simulink library "soar_interp"  (R2018b)
settings: Solver=VariableStepAuto  StartTime=0.0  StopTime=10.0  RelTol=1e-3
undefined symbols (not defined in the file): soarParams
settings Model: Creator=Taylor  LastModifiedBy=Nick's PC

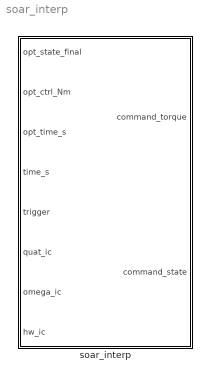
== system soar_interp ==
  soar_interp : Subsystem

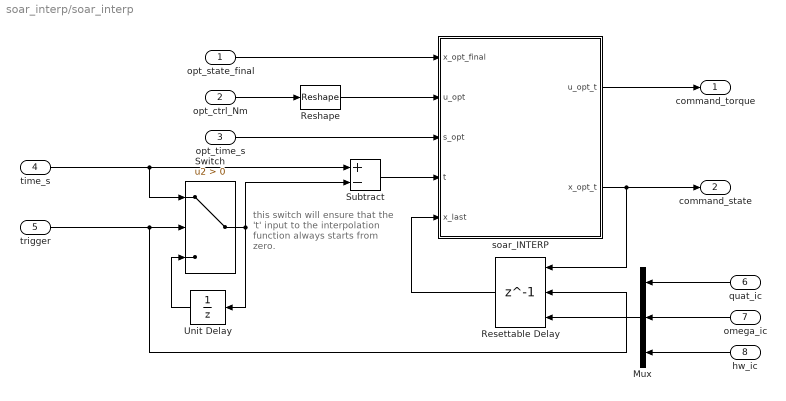
== system soar_interp/soar_interp ==
  note: this switch will ensure that the 't'
      | input to the interpolation function
      | always starts from zero.
  opt_state_final : Inport
  opt_ctrl_Nm : Inport  Port=2
  opt_time_s : Inport  Port=3
  time_s : Inport  Port=4
  trigger : Inport  Port=5
  quat_ic : Inport  Port=6
  omega_ic : Inport  Port=7
  hw_ic : Inport  Port=8
  Mux : Mux  Inputs=[4 3 3]
  Resettable Delay : Delay  DelayLength=1  InitialConditionSource=Input port  ExternalReset=Rising
      settings: InputPortMap=u0,r5,p4
  Reshape : Reshape  OutputDimensionality=Customize  OutputDimensions=[3,soarParams.N]
  Subtract : Sum  Inputs=+-
  Switch : Switch  Criteria=u2 > Threshold
  Unit Delay : UnitDelay  SampleTime=-1
  soar_INTERP : MATLAB Function  TreatAsAtomicUnit=on
  command_torque : Outport
  command_state : Outport  Port=2
  wires:
  omega_ic/1 -> Mux/2
  Mux/1 -> Resettable Delay/3
  Subtract/1 -> soar_INTERP/4(t)
  Resettable Delay/1 -> soar_INTERP/5(x_last)
  Unit Delay/1 -> Switch/3
  opt_state_final/1 -> soar_INTERP/1(x_opt_final)
  Switch/1 -> Unit Delay/1, Subtract/2
  Reshape/1 -> soar_INTERP/2(u_opt)
  trigger/1 -> Resettable Delay/2, Switch/2
  time_s/1 -> Switch/1, Subtract/1
  opt_ctrl_Nm/1 -> Reshape/1
  opt_time_s/1 -> soar_INTERP/3(s_opt)
  soar_INTERP/1(u_opt_t) -> command_torque/1
  soar_INTERP/2(x_opt_t) -> command_state/1, Resettable Delay/1
  quat_ic/1 -> Mux/1
  hw_ic/1 -> Mux/3

== matlab function soar_interp/soar_INTERP ==
  data: u_opt_t output size=3; x_opt_final input size=10; x_opt_t output size=10; u_opt input; s_opt input size=1; t input size=1; x_last input size=10; soarParams parameter
function [u_opt_t,x_opt_t] = soar_INTERP(x_opt_final,u_opt,s_opt,t,x_last,soarParams)
%SOAR_INTERP
%
% This function will interpolate the optimal solution from SOAR given the
% time t. Time t is assumed to represent the time SINCE the optimizer was
% called by flight software (necessitating the switch outside of this
% function). One RK4 step is performed to interpolate the state, while the
% control is interpolated using affine interpolation.
%
% T. Reynolds -- RAIN LAB

%#codegen

% parameters
N  = soarParams.N;
Ns = 10;
ut = linspace(0,s_opt,N);
k  = sum(t>ut); % current time interval
if (k==0); k = 1; end
J  = soarParams.inertia; % kg m2

% Output final state and ZERO feedforward control if we are beyond the 
% final maneuver time
if ((s_opt>eps)&&(t>=s_opt))
    u_opt_t = zeros(3,1);
    x_opt_t = [ x_opt_final(1:4); J\x_opt_final(5:7); x_opt_final(8:10) ];
    return;
end

% Otherwise integrate to current state and interpolate for current control
if ((k>0) && (s_opt>eps))
    dt = soarParams.sample_time_s/Ns;
    
    % step integrator for feedforward state x_opt_t
    x_opt_t = rk4_step(t,x_last,u_opt,ut,J,dt,Ns);

    % interpolate for feedforward control u_opt_t
    u_opt_t = zeros(3,1);
    for i = 1:3
        if t > ut(end) || t < ut(1)
            u_opt_t = zeros(3,1);
        else
            u_opt_t(i) = interp1(ut,u_opt(i,:),t,'linear');
        end
    end
else
    % this case happens when the optimizer has not yet been called
    u_opt_t = zeros(3,1);
    x_opt_t = x_last;
end

end % soar_interp

%%%%%%%%%%%%%%%%%%%%%%%%%%%%%%%%%%%%%%%%%%%%%%%%%%%%%%%%%%%%%%%%%%%%%%%%%%%
%%%%%%%%%%%%%%%%%%%%%%%%%%%% SUPPORT FUNCTIONS %%%%%%%%%%%%%%%%%%%%%%%%%%%%
%%%%%%%%%%%%%%%%%%%%%%%%%%%%%%%%%%%%%%%%%%%%%%%%%%%%%%%%%%%%%%%%%%%%%%%%%%%

function x = rk4_step(t,x,u,ut,J,h,Ns)

for ii = 1:Ns
    k1 = deriv(t     ,x      ,u,ut,J);
    k2 = deriv(t+h/2,x+h/2*k1,u,ut,J);
    k3 = deriv(t+h/2,x+h/2*k2,u,ut,J);
    k4 = deriv(t+h  ,x+h*k3  ,u,ut,J);

    x = (x + (h/6)*(k1+2*k2+2*k3+k4));
end

end

function dx = deriv(t,x,u,ut,J)
% Gives the *exact* same result when the momentum-based equations are used,
% this version is used here because the output needs to be angular velocity
% for FSW anyway.

% Divide by zero protection
mag = norm(x(1:4));
if mag < 1E-5 
    dx = zeros(size(x));
    return
end

% States
q   = x(1:4)./mag;

q0  = q(1);
qv  = q(2:4);
w   = x(5:7);
hw  = x(8:10);

% interpolate u_opt at time t
if t > ut(end) || t < ut(1)
    u_t = zeros(3,1);
else
    u_t = interp1(ut,u',t,'linear')';
end
% Kinematics & Dynamics
fq  = 0.5 * [ -qv'; skew(qv)+q0*eye(3) ] * w;
fw  = J\(-u_t - skew(w) * (J*w + hw));
fhw = u_t;

dx = [ fq; fw; fhw ];

end
